simulink model "experimenteren_deel_2"  (R2013a)
settings: Solver=FixedStepDiscrete  StartTime=0.0  StopTime=200  FixedStep=1/44100  RelTol=1e-3
InitFcn:
  | input_frame_size = 4096;
  | frame_size = 4096;
  | overlap = 0.5;
  | alpha = 1.5;
  | 
  | k = round(frame_size - alpha*(1-overlap)*frame_size);
libraries: dspmtrx3 x4, dspsigops x1, dspsrcs4 x1, dspsnks4 x1
settings Model: Creator=Tomas  LastModifiedBy=Tomas

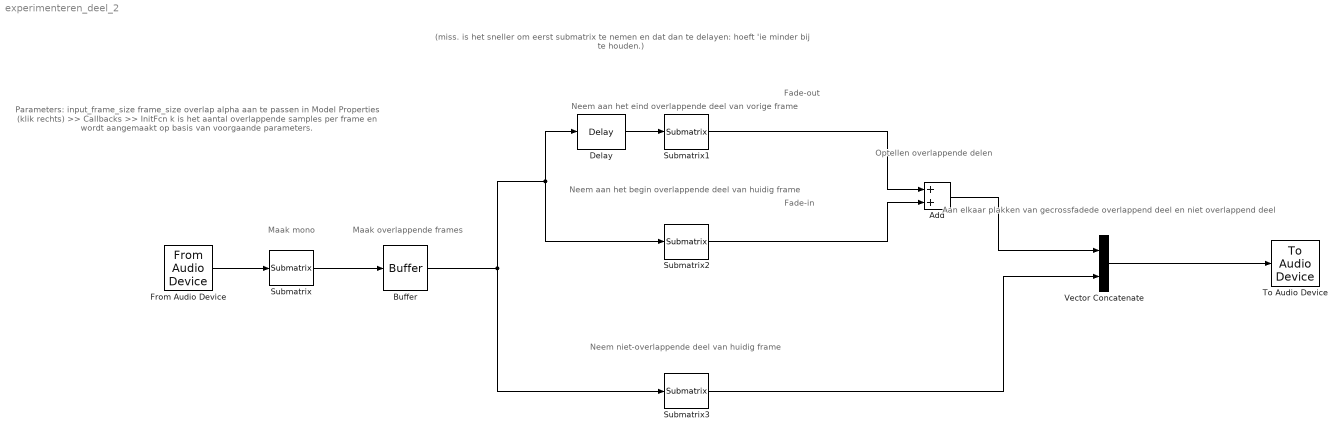
== system experimenteren_deel_2 ==
  note: (miss. is het sneller om eerst submatrix te nemen
      | en dat dan te delayen: hoeft 'ie minder bij te houden.)
  note: Aan elkaar plakken van
      | gecrossfadede overlappend deel
      | en niet overlappend deel
  note: Optellen
      | overlappende delen
  note: Neem niet-overlappende deel
      | van huidig frame
  note: Fade-in
  note: Fade-out
  note: Neem aan het begin overlappende
      | deel van huidig frame
  note: Neem aan het eind overlappende
      | deel van vorige frame
  note: Parameters:
      | input_frame_size
      | frame_size
      | overlap
      | alpha
      |
      | aan te passen in
      |
      | Model Properties (klik rechts)
      |  >> Callbacks >> InitFcn
      |
      | k is het aantal overlappende
      |  samples per frame en wordt
      | aangemaakt op basis van
      | voorgaande parameters.
  note: Maak overlappende frames
  note: Maak mono
  Add : Sum  Inputs=2
  Buffer : Buffer  N=frame_size  V=round(frame_size*overlap)  TreatMby1Signals=One channel
  Delay : dspsigops/Delay  InputProcessing=Columns as channels (frame based)  dly_unit=Frames  delay=1  ic_detail=off  dif_ic_for_ch=off  dif_ic_for_dly=off  ic=0  reset_popup=None
  From Audio Device : dspsrcs4/From Audio Device  deviceName=Default  numChannels=1  sampleRate=44100  deviceDatatype=Determine from output data type  autoBufferSize=on  bufferSize=4096  queueDuration=0  frameSize=input_frame_size  outputDatatype=single
  Submatrix : dspmtrx3/Submatrix  RowSpan=All rows  RowStartMode=First  RowStartIndex=1  RowEndMode=Last  RowEndIndex=1  ColSpan=One column  ColStartMode=First  ColStartIndex=1  ColEndMode=Last  ColEndIndex=1
  Submatrix1 : dspmtrx3/Submatrix  RowSpan=Range of rows  RowStartMode=Offset from last  RowStartIndex=k-1  RowEndMode=Last  RowEndIndex=1  ColSpan=All columns  ColStartMode=Offset from last  ColStartIndex=k  ColEndMode=Last  ColEndIndex=1
  Submatrix2 : dspmtrx3/Submatrix  RowSpan=Range of rows  RowStartMode=First  RowStartIndex=1  RowEndMode=Index  RowEndIndex=k  ColSpan=All columns  ColStartMode=Offset from last  ColStartIndex=k  ColEndMode=Last  ColEndIndex=1
  Submatrix3 : dspmtrx3/Submatrix  RowSpan=Range of rows  RowStartMode=Index  RowStartIndex=k+1  RowEndMode=Offset from last  RowEndIndex=k  ColSpan=All columns  ColStartMode=Offset from last  ColStartIndex=k  ColEndMode=Last  ColEndIndex=1
  To Audio Device : dspsnks4/To Audio Device  deviceName=Default  inheritSampleRate=on  sampleRate=44100  deviceDatatype=Determine from input data type  autoBufferSize=on  bufferSize=4096  queueDuration=0
  Vector Concatenate : Concatenate  Mode=Multidimensional array
  wires:
  From Audio Device/1 -> Submatrix/1
  Submatrix/1 -> Buffer/1
  Buffer/1 -> Submatrix2/1, Delay/1, Submatrix3/1
  Delay/1 -> Submatrix1/1
  Submatrix2/1 -> Add/2
  Add/1 -> Vector Concatenate/1
  Submatrix3/1 -> Vector Concatenate/2
  Vector Concatenate/1 -> To Audio Device/1
  Submatrix1/1 -> Add/1
